simulink library "ctp"  (Simulink 8.2)
settings: Solver=ode1  StartTime=0.0  StopTime=Inf  FixedStep=0.001  RelTol=1e-3
PostLoadFcn:
  | , if any(exist('dsrtsu_mdlpostloadfcn', 'file') == [2, 3, 6]), try dsrtsu_mdlpostloadfcn('Execute', bdroot); catch fprintf('Error in PostLoadFcn (dsrtsu_mdlpostloadfcn) for model "%s":\n %s\n', bdroot, lasterr); end, end,
undefined symbols (not defined in the file or in its folder): AACC_ACCVehSpdTqMap_kph, AACC_DesiredDistMap_m, FALSE, KACC_ACCTqControllerKdMap_flg, KACC_ACCTqErrorGParam_num, KACC_ACCTqFFParam_num, KACC_ACCTqInitialIParam_num, KACC_ACCTqKdFixedGain_num, KACC_ACCTqKdGain_num, KACC_ACCTqKiGain_num, KACC_ACCTqKpGain_num, KACC_ACCTqMaxIParam_num, KACC_ACCTqMinIParam_num, KACC_ACCTqResetIParam_num, MACC_TorquePIDDistErrorG_num, MACC_TorquePIDErrorG_num, MACC_TorquePIDKd_num, MACC_TorquePIDKp_num, MPS2KPH
libraries: hcu_lib x7
settings Model: DSRTSU_INTERNAL_RTI_VER=450  DSRTSU_INTERNAL_RTI_TYPE=rti1401  RTICANMMDATA=struct('GeneralSetupData',struct('modelroot','D:\ActiveSafetyDepartment\SVN\trunk\ADAS_Softwares\HTDragon\software\sw_development\arch\app\acc','generalsettings',struct('filesettings',struct('destfolder',struct('Name','RTICANMM_FILES','Check',1),'buildfolder',struct('Name','.','Check',1),'AbsDestfolder',struct('Name','D:\ActiveSafetyDepartment\SVN\trunk\ADAS_Softwares\HTDragon\software\sw_development\arch\app\acc\RTICANMM_FILES'),'AbsBuildfolder',struct('Name','D:\ActiveSafetyDepartment\SVN\trunk\ADAS_Softwares\HTDragon\software\sw_development\arch\app\acc'))),'options',struct('addpaths',1,'rmpaths',1,'addtrcexclusion',logical(1),'cannavigator',struct('checkmonitoring',0),'show_usrtrc',0,'use_usrtrc',0),'advanced',struct('options',[1 1 1 1 1 1 1 1 1 1 1 1 1 1 1 1 1 1 1 1 1 1 1 1 1 1 1 1 1 1 1 1 1 1 1 1 1 1 1 1 1 1 1 1 1 1 1 1 1 1 1 1 1 1 1 1 1 1 1 1 1 1 1 1 1 1 1 1 1 1 1 1 1 1 1 1 1 1 1 1 1 1 1 1 1 1 1 1 1 1 1 1 1 1 1 1 1 1 1 1]),'MPSetup',{{}},'modelname','ctp','block','ctp'))  DSRTSU_INTERNAL_RTIFPGA=40  Creator=AT015411  LastModifiedBy=14069

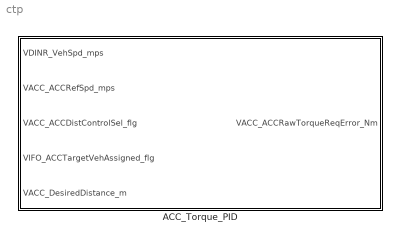
== system ctp ==
  ACC_Torque_PID : Subsystem

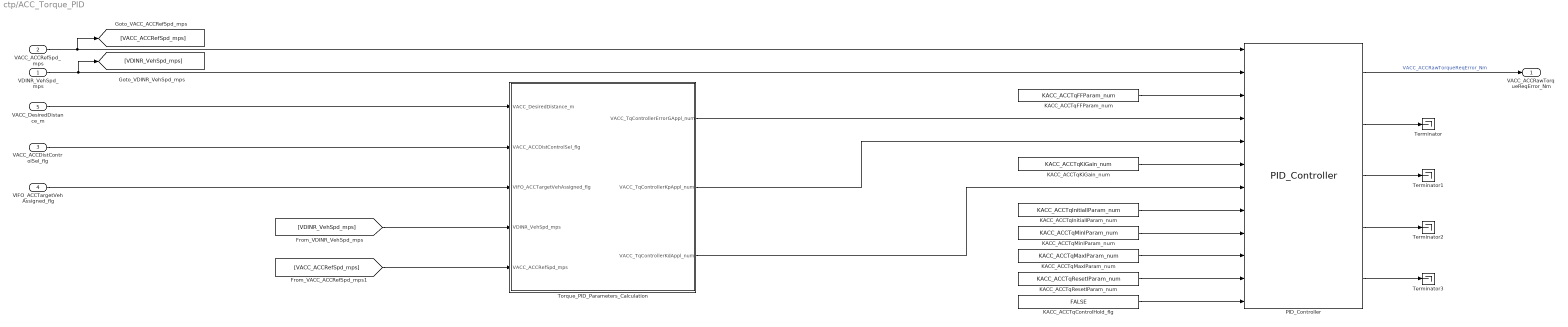
== system ctp/ACC_Torque_PID ==
  VDINR_VehSpd_mps : Inport
  VACC_ACCRefSpd_mps : Inport  Port=2
  VACC_ACCDistControlSel_flg : Inport  Port=3
  VIFO_ACCTargetVehAssigned_flg : Inport  Port=4
  VACC_DesiredDistance_m : Inport  Port=5
  KACC_ACCTqControlHold_flg : Constant  Value=FALSE  OutDataTypeStr=boolean
  KACC_ACCTqFFParam_num : Constant  Value=KACC_ACCTqFFParam_num
  KACC_ACCTqInitialIParam_num : Constant  Value=KACC_ACCTqInitialIParam_num
  KACC_ACCTqKiGain_num : Constant  Value=KACC_ACCTqKiGain_num
  KACC_ACCTqMaxIParam_num : Constant  Value=KACC_ACCTqMaxIParam_num
  KACC_ACCTqMinIParam_num : Constant  Value=KACC_ACCTqMinIParam_num
  KACC_ACCTqResetIParam_num : Constant  Value=KACC_ACCTqResetIParam_num
  PID_Controller : hcu_lib/PID_Controller  SystemSampleTime=-1
  Terminator{,1..3} (4 alike) : Terminator
  Torque_PID_Parameters_Calculation : Subsystem
  VACC_ACCRawTorqueReqError_Nm : Outport
  wires:
  KACC_ACCTqControlHold_flg/1 -> PID_Controller/12
  PID_Controller/5 -> Terminator3/1
  VDINR_VehSpd_mps/1 -> [VDINR_VehSpd_mps], PID_Controller/2
  KACC_ACCTqMinIParam_num/1 -> PID_Controller/9
  KACC_ACCTqMaxIParam_num/1 -> PID_Controller/10
  KACC_ACCTqInitialIParam_num/1 -> PID_Controller/8
  KACC_ACCTqFFParam_num/1 -> PID_Controller/3
  KACC_ACCTqResetIParam_num/1 -> PID_Controller/11
  PID_Controller/3 -> Terminator1/1
  PID_Controller/2 -> Terminator/1
  PID_Controller/4 -> Terminator2/1
  VACC_ACCRefSpd_mps/1 -> [VACC_ACCRefSpd_mps], PID_Controller/1
  PID_Controller/1 -> VACC_ACCRawTorqueReqError_Nm/1  "VACC_ACCRawTorqueReqError_Nm"
  KACC_ACCTqKiGain_num/1 -> PID_Controller/6
  VACC_DesiredDistance_m/1 -> Torque_PID_Parameters_Calculation/1(VACC_DesiredDistance_m)
  VACC_ACCDistControlSel_flg/1 -> Torque_PID_Parameters_Calculation/2(VACC_ACCDistControlSel_flg)
  VIFO_ACCTargetVehAssigned_flg/1 -> Torque_PID_Parameters_Calculation/3(VIFO_ACCTargetVehAssigned_flg)
  Torque_PID_Parameters_Calculation/1(VACC_TqControllerErrorGAppl_num) -> PID_Controller/4
  Torque_PID_Parameters_Calculation/2(VACC_TqControllerKpAppl_num) -> PID_Controller/5
  Torque_PID_Parameters_Calculation/3(VACC_TqControllerKdAppl_num) -> PID_Controller/7
  [VACC_ACCRefSpd_mps] -> Torque_PID_Parameters_Calculation/5(VACC_ACCRefSpd_mps)
  [VDINR_VehSpd_mps] -> Torque_PID_Parameters_Calculation/4(VDINR_VehSpd_mps)

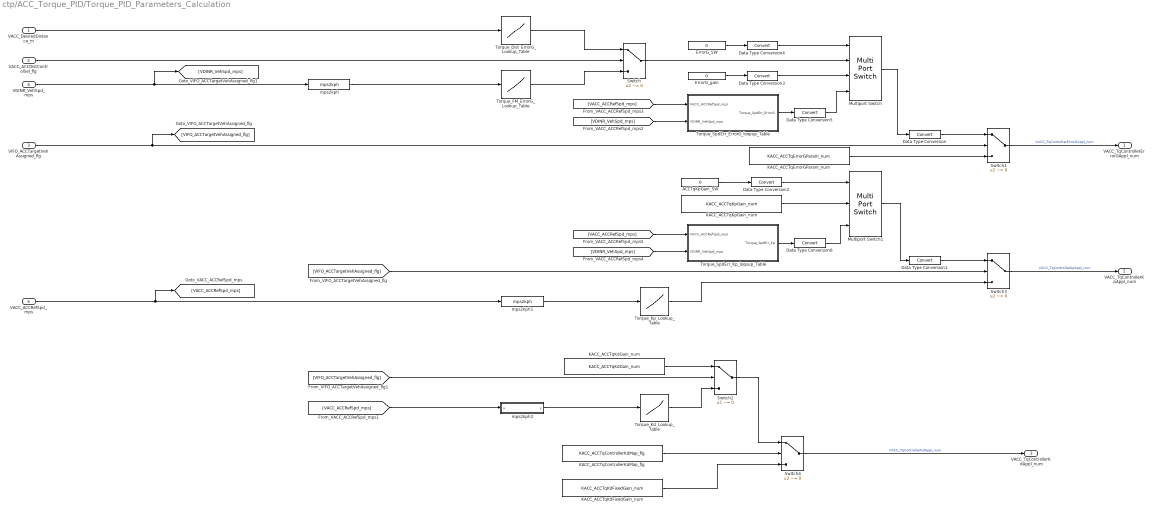
== system ctp/ACC_Torque_PID/Torque_PID_Parameters_Calculation ==
  VACC_DesiredDistance_m : Inport
  VACC_ACCDistControlSel_flg : Inport  Port=2
  VIFO_ACCTargetVehAssigned_flg : Inport  Port=3
  VDINR_VehSpd_mps : Inport  Port=4
  VACC_ACCRefSpd_mps : Inport  Port=5
  ACCTqKpGain_SW : Constant  Value=0
  Data Type Conversion{,1..6} (7 alike) : DataTypeConversion
  ErrorG_SW : Constant  Value=0
  ErrorG_gain : Constant  Value=0
  KACC_ACCTqControllerKdMap_flg : Constant  Value=KACC_ACCTqControllerKdMap_flg
  KACC_ACCTqErrorGParam_num : Constant  Value=KACC_ACCTqErrorGParam_num
  KACC_ACCTqKdFixedGain_num : Constant  Value=KACC_ACCTqKdFixedGain_num
  KACC_ACCTqKdGain_num : Constant  Value=KACC_ACCTqKdGain_num
  KACC_ACCTqKpGain_num : Constant  Value=KACC_ACCTqKpGain_num
  Multiport Switch : MultiPortSwitch  DataPortOrder=Zero-based contiguous
  Multiport Switch1 : MultiPortSwitch  DataPortOrder=Zero-based contiguous  Inputs=2
  Switch{,1..4} (5 alike) : Switch  Criteria=u2 ~= 0
  Torque_Dist_ErrorG_Lookup_Table : Lookup_n-D  NumberOfTableDimensions=1  BreakpointsForDimension1=AACC_DesiredDistMap_m  Table=MACC_TorquePIDDistErrorG_num  ExtrapMethod=Clip  UseLastTableValue=on  RndMeth=Simplest  InputSameDT=on
  Torque_FM_ErrorG_Lookup_Table : Lookup_n-D  NumberOfTableDimensions=1  BreakpointsForDimension1=AACC_ACCVehSpdTqMap_kph  Table=MACC_TorquePIDErrorG_num  ExtrapMethod=Clip  UseLastTableValue=on  RndMeth=Simplest  InputSameDT=on
  Torque_Kd_Lookup_Table : Lookup_n-D  NumberOfTableDimensions=1  BreakpointsForDimension1=AACC_ACCVehSpdTqMap_kph  Table=MACC_TorquePIDKd_num  ExtrapMethod=Clip  UseLastTableValue=on  RndMeth=Simplest  InputSameDT=on
  Torque_Kp_Lookup_Table : Lookup_n-D  NumberOfTableDimensions=1  BreakpointsForDimension1=AACC_ACCVehSpdTqMap_kph  Table=MACC_TorquePIDKp_num  ExtrapMethod=Clip  UseLastTableValue=on  RndMeth=Simplest  InputSameDT=on
  Torque_SpdErr_ErrorG_loopup_Table : Subsystem
  Torque_SpdErr_Kp_loopup_Table : Subsystem
  mps2kph : hcu_lib/mps2kph
  mps2kph1 : hcu_lib/mps2kph
  mps2kph2 : Subsystem  mask(Conversion){}
      mask help: Convert Meters per second to Kilometers per hour
      mask Display: disp('m/s \rightarrow km/h', 'texmode', 'on')
  VACC_TqControllerErrorGAppl_num : Outport
  VACC_TqControllerKpAppl_num : Outport  Port=2
  VACC_TqControllerKdAppl_num : Outport  Port=3
  wires:
  Switch1/1 -> VACC_TqControllerErrorGAppl_num/1  "VACC_TqControllerErrorGAppl_num"
  VACC_ACCDistControlSel_flg/1 -> Switch/2
  VIFO_ACCTargetVehAssigned_flg/1 -> [VIFO_ACCTargetVehAssigned_flg], Switch1/2
  KACC_ACCTqErrorGParam_num/1 -> Switch1/3
  Multiport Switch1/1 -> Data Type Conversion1/1
  Multiport Switch/1 -> Data Type Conversion/1
  mps2kph1/1 -> Torque_Kp_Lookup_Table/1
  Torque_Kp_Lookup_Table/1 -> Switch3/3
  VACC_DesiredDistance_m/1 -> Torque_Dist_ErrorG_Lookup_Table/1
  [VIFO_ACCTargetVehAssigned_flg] -> Switch3/2
  Switch3/1 -> VACC_TqControllerKpAppl_num/1  "VACC_TqControllerKpAppl_num"
  VDINR_VehSpd_mps/1 -> [VDINR_VehSpd_mps], mps2kph/1
  Torque_Dist_ErrorG_Lookup_Table/1 -> Switch/1
  mps2kph/1 -> Torque_FM_ErrorG_Lookup_Table/1
  mps2kph2/1(y) -> Torque_Kd_Lookup_Table/1
  Torque_FM_ErrorG_Lookup_Table/1 -> Switch/3
  Torque_Kd_Lookup_Table/1 -> Switch2/3
  KACC_ACCTqKdGain_num/1 -> Switch2/1
  [VACC_ACCRefSpd_mps] -> mps2kph2/1(u)
  [VIFO_ACCTargetVehAssigned_flg] -> Switch2/2
  Switch4/1 -> VACC_TqControllerKdAppl_num/1  "VACC_TqControllerKdAppl_num"
  Switch2/1 -> Switch4/1
  KACC_ACCTqKdFixedGain_num/1 -> Switch4/3
  KACC_ACCTqControllerKdMap_flg/1 -> Switch4/2
  VACC_ACCRefSpd_mps/1 -> mps2kph1/1, [VACC_ACCRefSpd_mps]
  Switch/1 -> Multiport Switch/2
  ErrorG_SW/1 -> Data Type Conversion4/1
  ErrorG_gain/1 -> Data Type Conversion3/1
  [VACC_ACCRefSpd_mps] -> Torque_SpdErr_ErrorG_loopup_Table/1(VACC_ACCRefSpd_mps)
  [VDINR_VehSpd_mps] -> Torque_SpdErr_ErrorG_loopup_Table/2(VDINR_VehSpd_mps)
  Torque_SpdErr_ErrorG_loopup_Table/1(Torque_SpdErr_ErrorG) -> Data Type Conversion5/1
  KACC_ACCTqKpGain_num/1 -> Multiport Switch1/2
  ACCTqKpGain_SW/1 -> Data Type Conversion2/1
  [VACC_ACCRefSpd_mps] -> Torque_SpdErr_Kp_loopup_Table/1(VACC_ACCRefSpd_mps)
  [VDINR_VehSpd_mps] -> Torque_SpdErr_Kp_loopup_Table/2(VDINR_VehSpd_mps)
  Torque_SpdErr_Kp_loopup_Table/1(Torque_SpdErr_Kp) -> Data Type Conversion6/1
  Data Type Conversion/1 -> Switch1/1
  Data Type Conversion1/1 -> Switch3/1
  Data Type Conversion2/1 -> Multiport Switch1/1
  Data Type Conversion3/1 -> Multiport Switch/3
  Data Type Conversion4/1 -> Multiport Switch/1
  Data Type Conversion5/1 -> Multiport Switch/4
  Data Type Conversion6/1 -> Multiport Switch1/3

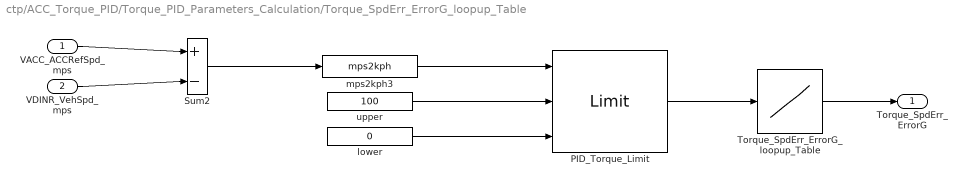
== system ctp/ACC_Torque_PID/Torque_PID_Parameters_Calculation/Torque_SpdErr_ErrorG_loopup_Table ==
  VACC_ACCRefSpd_mps : Inport
  VDINR_VehSpd_mps : Inport  Port=2
  PID_Torque_Limit : hcu_lib/Limit  SystemSampleTime=-1
  Sum2 : Sum  Inputs=+|-  SaturateOnIntegerOverflow=on  InputSameDT=on  OutDataTypeStr=Inherit: Same as first input
  Torque_SpdErr_ErrorG_loopup_Table : Lookup_n-D  NumberOfTableDimensions=1  BreakpointsForDimension1=[0 5 10 15 20 25 30 35 40 45 50 55 60 65 70 75]  Table=[0 0.1 0.2 1 1 1 1 1 1 1 1 1 1 1 1 1]  InternalRulePriority=Speed  RndMeth=Simplest  InputSameDT=on
  lower : Constant  Value=0
  mps2kph3 : hcu_lib/mps2kph
  upper : Constant  Value=100
  Torque_SpdErr_ErrorG : Outport
  wires:
  VDINR_VehSpd_mps/1 -> Sum2/2
  VACC_ACCRefSpd_mps/1 -> Sum2/1
  Sum2/1 -> mps2kph3/1
  mps2kph3/1 -> PID_Torque_Limit/1
  Torque_SpdErr_ErrorG_loopup_Table/1 -> Torque_SpdErr_ErrorG/1
  PID_Torque_Limit/1 -> Torque_SpdErr_ErrorG_loopup_Table/1
  upper/1 -> PID_Torque_Limit/2
  lower/1 -> PID_Torque_Limit/3

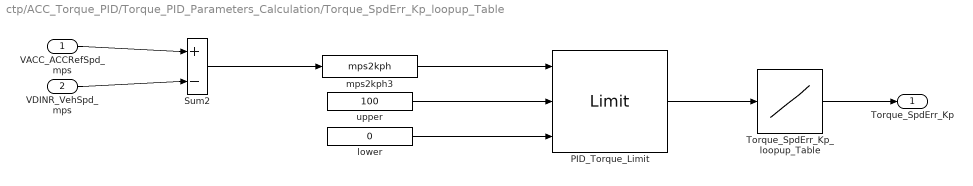
== system ctp/ACC_Torque_PID/Torque_PID_Parameters_Calculation/Torque_SpdErr_Kp_loopup_Table ==
  VACC_ACCRefSpd_mps : Inport
  VDINR_VehSpd_mps : Inport  Port=2
  PID_Torque_Limit : hcu_lib/Limit  SystemSampleTime=-1
  Sum2 : Sum  Inputs=+|-  SaturateOnIntegerOverflow=on  InputSameDT=on  OutDataTypeStr=Inherit: Same as first input
  Torque_SpdErr_Kp_loopup_Table : Lookup_n-D  NumberOfTableDimensions=1  BreakpointsForDimension1=[0 5 10 15 20 25 30 35 40 45 50 55 60 65 70 75]  Table=[0 10 15 20 25 30 35 40 45 50 55 60 65 70 75 80]  InternalRulePriority=Speed  RndMeth=Simplest  InputSameDT=on
  lower : Constant  Value=0
  mps2kph3 : hcu_lib/mps2kph
  upper : Constant  Value=100
  Torque_SpdErr_Kp : Outport
  wires:
  VDINR_VehSpd_mps/1 -> Sum2/2
  VACC_ACCRefSpd_mps/1 -> Sum2/1
  Sum2/1 -> mps2kph3/1
  mps2kph3/1 -> PID_Torque_Limit/1
  Torque_SpdErr_Kp_loopup_Table/1 -> Torque_SpdErr_Kp/1
  PID_Torque_Limit/1 -> Torque_SpdErr_Kp_loopup_Table/1
  upper/1 -> PID_Torque_Limit/2
  lower/1 -> PID_Torque_Limit/3

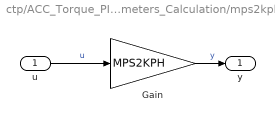
== system ctp/ACC_Torque_PID/Torque_PID_Parameters_Calculation/mps2kph2 ==
  u : Inport
  Gain : Gain  Gain=MPS2KPH
  y : Outport
  wires:
  u/1 -> Gain/1  "u"
  Gain/1 -> y/1  "y"
